simulink model "complementary_filter"  (Simulink 7.4)
settings: Solver=FixedStepDiscrete  StartTime=0.0  StopTime=10  RelTol=1e-3
values from neighbouring files (symbols this model uses):
  g = 9.81    [complementary_filter_param.m]    (also in quadrocopter_param.m)
  HPF = 0.95    [complementary_filter_param.m]    (also in quadrocopter_param.m)
  LPF = 0.05    [complementary_filter_param.m]    (also in quadrocopter_param.m)
  Ts = 0.01    [complementary_filter_param.m]    (also in quadrocopter_param.m)
libraries: simulink x2
settings Model: Creator=Sreekanth  LastModifiedBy=Sreekanth
settings DebuggingCC: AlgebraicLoopMsg=none

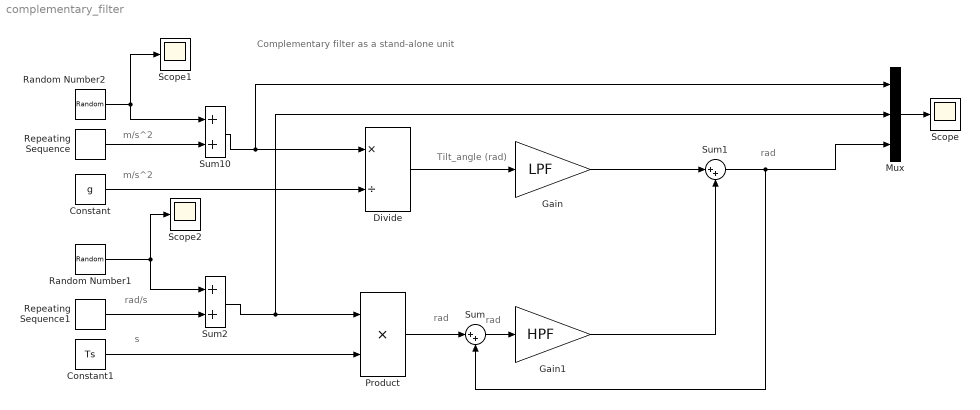
== system complementary_filter ==
  note: Tilt_angle (rad)
  note: m/s^2
  note: m/s^2
  note: rad/s
  note: s
  note: rad
  note: rad
  note: rad
  note: Complementary filter as a stand-alone unit
  Constant : Constant  Value=g  OutDataType=fixdt(1, 16)  OutScaling=2^0  SampleTime=Ts
  Constant1 : Constant  Value=Ts  OutDataType=fixdt(1, 16)  OutScaling=2^0  SampleTime=Ts
  Divide : Product  Inputs=*/  OutDataType=fixdt(1, 16)  OutScaling=2^-10
  Gain : Gain  Gain=LPF  ParameterDataType=fixdt(1, 16)  ParameterScaling=2^0  OutDataType=fixdt(1, 16)  OutScaling=2^0  SampleTime=Ts
  Gain1 : Gain  Gain=HPF  ParameterDataType=fixdt(1, 16)  ParameterScaling=2^0  OutDataType=fixdt(1, 16)  OutScaling=2^0  SampleTime=Ts
  Mux : Mux  Inputs=3
  Product : Product  OutDataType=fixdt(1, 16)  OutScaling=2^0  RndMeth=Zero
  Random Number1 : RandomNumber  Variance=0.05  SampleTime=Ts
  Random Number2 : RandomNumber  Variance=0.05  SampleTime=Ts
  Repeating Sequence : simulink/Sources/Repeating Sequence  SystemSampleTime=-1  rep_seq_t=[0 1 2 3 4 5 6 7 8 9 10]  rep_seq_y=[0.2 0.6 0.4 0.5 0.4 0.5 0.4 0.5 0.4 0.5 0.5]
  Repeating Sequence1 : simulink/Sources/Repeating Sequence  SystemSampleTime=-1  rep_seq_t=[0 1 2 3 4 5 6 7 8 9 10]  rep_seq_y=[0.1 0.3 0.2 0.2 0.2 0.3 0.3 0.4 0.2 0.2 0.2]
  Scope : Scope
      settings: YMin=0  YMax=1
  Scope1 : Scope
      settings: YMin=0  YMax=1
  Scope2 : Scope
      settings: YMin=0  YMax=1  SaveName=ScopeData2
  Sum : Sum  Inputs=|++  OutDataType=fixdt(1, 16)  OutScaling=2^0
  Sum1 : Sum  Inputs=|++  OutDataType=fixdt(1, 16)  OutScaling=2^0
  Sum10 : Sum  OutDataType=fixdt(1, 16)  OutScaling=2^0
  Sum2 : Sum  OutDataType=fixdt(1, 16)  OutScaling=2^0
  wires:
  Constant/1 -> Divide/2
  Divide/1 -> Gain/1
  Constant1/1 -> Product/2
  Product/1 -> Sum/1
  Gain/1 -> Sum1/1
  Gain1/1 -> Sum1/2
  Sum1/1 -> Sum/2, Mux/3
  Sum/1 -> Gain1/1
  Mux/1 -> Scope/1
  Random Number2/1 -> Sum10/1, Scope1/1
  Repeating Sequence/1 -> Sum10/2
  Sum10/1 -> Divide/1, Mux/1
  Random Number1/1 -> Sum2/1, Scope2/1
  Repeating Sequence1/1 -> Sum2/2
  Sum2/1 -> Product/1, Mux/2
